simulink library "Tower"  (Simulink 7.9)
settings: Solver=ode45  StartTime=0.0  StopTime=10.0  RelTol=1e-3
undefined symbols (not defined in the file): WT_Params
libraries: mblibv1 x3
Description:
  | Copyright 2011 MathWorks, Inc.
settings Model: Creator=smiller  LastModifiedBy=smiller

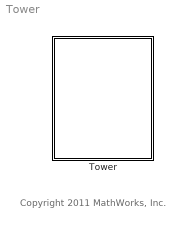
== system Tower ==
  note: Copyright 2011 MathWorks, Inc.
  Tower : Subsystem
      mask Display:
      | image(imread('Tower_IMAGE.jpg'));
      | port_label('RConn',1,'Env');
      | port_label('RConn',2,'GrVa');
      | port_label('RConn',3,'GrVb');
      | port_label('RConn',4,'GrVc');
      | port_label('LConn',1,'N');
      | port_label('LConn',2,'GrVa');
      | port_label('LConn',3,'GrVb');
      | port_label('LConn',4,'GrVc');

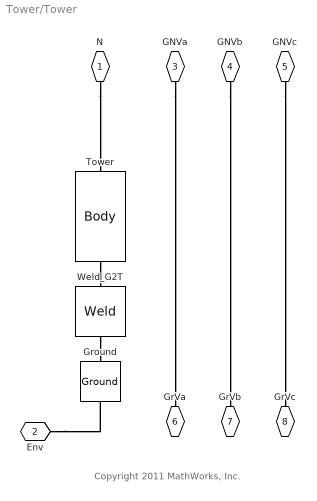
== system Tower/Tower ==
  note: Copyright 2011 MathWorks, Inc.
  Ground : mblibv1/Bodies/Ground  UpdateFromCAD=off  LeftPortType=env  RightPortType=workingframe  PhysicalDomain=Mechanical  DialogClass=GroundBlock  CoordPosition=[0 0 0]  CoordPositionUnits=m  StateVectorMgrId=-1  MachineId=[0 0]  ShowEnvPort=on
  Tower : mblibv1/Bodies/Body  LConnTagsString=CS1  RConnTagsString=CS2  UpdateFromCAD=off  DialogClass=MechanicalBodyBlock  Mass=WT_Params.Tower.mass  MassUnits=kg  InertiaUnits=kg*m^2  Inertia=WT_Params.Tower.inertia  Shape=Cylinder  ShapeDims=[1 1]  ShapeUnits=m  ShapeUse=false  Density=1  DensityUnits=kg/m^3  DensityUse=false  GraphicsMode=MACHINE_DEFAULT  BodyColorSelMode=COLORPALETTE  BodyColor=[1 1 1]  AttachedToCS=CG  CG=Left$CG$[0 0 0]$CS1$CS1$m$[0 0 0]$Euler X-Y-Z$deg$ADJOINING$false$none  WorkingFrames=Left$CS1$[0 0 0]$Adjoining$Adjoining$m$[0 0 0]$Euler X-Y-Z$deg$CG$true$none#Right$CS2$[0 WT_Params.Tower.height 0]$CS1$CS1$m$[0 0 0]$Euler X-Y-Z$deg$CG$true$none#Right$CS5$[0 0 0]$CG$CG$m$[0 0 0]$Euler X-Y-Z$deg$CG$false$none#Right$CS7$[WT_Params.Tower.base_radius*cos(0) 0 WT_Params.Tower.base_radius*sin(0)]$CG$CG$m$[0 0 0]$Euler X-Y-Z$deg$CG$false$none#Right$CS8$[WT_Params.Tower.base_radius*cos(0.2*pi) 0 WT_Params.Tower.base_radius*sin(0.2*pi)]$CG$CG$m$[0 0 0]$Euler X-Y-Z$deg$CG$false$none#Right$CS9$[WT_Params.Tower.base_radius*cos(0.4*pi) 0 WT_Params.Tower.base_radius*sin(0.4*pi)]$CG$CG$m$[0 0 0]$Euler X-Y-Z$deg$CG$false$none#Right$CS10$[WT_Params.Tower.base_radius*cos(0.6*pi) 0 WT_Params.Tower.base_radius*sin(0.6*pi)]$CG$CG$m$[0 0 0]$Euler X-Y-Z$deg$CG$false$none#Right$CS11$[WT_Params.Tower.base_radius*cos(0.8*pi) 0 WT_Params.Tower.base_radius*sin(0.8*pi)]$CG$CG$m$[0 0 0]$Euler X-Y-Z$deg$CG$false$none#Right$CS12$[WT_Params.Tower.base_radius*cos(1.0*pi) 0 WT_Params.Tower.base_radius*sin(1.0*pi)]$CG$CG$m$[0 0 0]$Euler X-Y-Z$deg$CG$false$none#Right$CS13$[WT_Params.Tower.base_radius*cos(1.2*pi) 0 WT_Params.Tower.base_radius*sin(1.2*pi)]$CG$CG$m$[0 0 0]$Euler X-Y-Z$deg$CG$false$none#Right$CS14$[WT_Params.Tower.base_radius*cos(1.4*pi) 0 WT_Params.Tower.base_radius*sin(1.4*pi)]$CG$CG$m$[0 0 0]$Euler X-Y-Z$deg$CG$false$none#Right$CS15$[WT_Params.Tower.base_radius*cos(1.6*pi) 0 WT_Params.Tower.base_radius*sin(1.6*pi)]$CG$CG$m$[0 0 0]$Euler X-Y-Z$deg$CG$false$none#Right$CS16$[WT_Params.Tower.base_radius*cos(1.8*pi) 0 WT_Params.Tower.base_radius*sin(1.8*pi)]$CG$CG$m$[0 0 0]$Euler X-Y-Z$deg$CG$false$none#Right$CS17$[WT_Params.Tower.top_radius*cos(0) WT_Params.Tower.height WT_Params.Tower.top_radius*sin(0)]$CG$CG$m$[0 0 0]$Euler X-Y-Z$deg$CG$false$none#Right$CS18$[WT_Params.Tower.top_radius*cos(0.2*pi) WT_Params.Tower.height WT_Params.Tower.top_radius*sin(0.2*pi)]$CG$CG$m$[0 0 0]$Euler X-Y-Z$deg$CG$false$none#Right$CS19$[WT_Params.Tower.top_radius*cos(0.4*pi) WT_Params.Tower.height WT_Params.Tower.top_radius*sin(0.4*pi)]$CG$CG$m$[0 0 0]$Euler X-Y-Z$deg$CG$false$none#Right$CS20$[WT_Params.Tower.top_radius*cos(0.6*pi) WT_Params.Tower.height WT_Params.Tower.top_radius*sin(0.6*pi)]$CG$CG$m$[0 0 0]$Euler X-Y-Z$deg$CG$false$none#Right$CS21$[WT_Params.Tower.top_radius*cos(0.8*pi) WT_Params.Tower.height WT_Params.Tower.top_radius*sin(0.8*pi)]$CG$CG$m$[0 0 0]$Euler X-Y-Z$deg$CG$false$none#Right$CS22$[WT_Params.Tower.top_radius*cos(1.0*pi) WT_Params.Tower.height WT_Params.Tower.top_radius*sin(1.0*pi)]$CG$CG$m$[0 0 0]$Euler X-Y-Z$deg$CG$false$none#Right$CS23$[WT_Params.Tower.top_radius*cos(1.2*pi) WT_Params.Tower.height WT_Params.Tower.top_radius*sin(1.2*pi)]$CG$CG$m$[0 0 0]$Euler X-Y-Z$deg$CG$false$none#Right$CS24$[WT_Params.Tower.top_radius*cos(1.4*pi) WT_Params.Tower.height WT_Params.Tower.top_radius*sin(1.4*pi)]$CG$CG$m$[0 0 0]$Euler X-Y-Z$deg$CG$false$none#Right$CS25$[WT_Params.Tower.top_radius*cos(1.6*pi) WT_Params.Tower.height WT_Params.Tower.top_radius*sin(1.6*pi)]$CG$CG$m$[0 0 0]$Euler X-Y-Z$deg$CG$false$none#Right$CS26$[WT_Params.Tower.top_radius*cos(1.8*pi) WT_Params.Tower.height WT_Params.Tower.top_radius*sin(1.8*pi)]$CG$CG$m$[0 0 0]$Euler X-Y-Z$deg$CG$false$none  CGPos=[0 0 0]  CGRot=[0 0 0]  CS0Pos=[]  CS0Rot=[]  CS1Pos=[0 0 0]  CS1Rot=[0 0 0]  CS2Pos=[0 WT_Params.Tower.height 0]  CS2Rot=[0 0 0]  CS3Pos=[]  CS3Rot=[]  CS4Pos=[]  CS4Rot=[]  CS5Pos=[0 0 0]  CS5Rot=[0 0 0]  CS6Pos=[]  CS6Rot=[]  CS7Pos=[WT_Params.Tower.base_radius*cos(0) 0 WT_Params.Tower.base_radius*sin(0)]  CS7Rot=[0 0 0]  CS8Pos=[WT_Params.Tower.base_radius*cos(0.2*pi) 0 WT_Params.Tower.base_radius*sin(0.2*pi)]  CS8Rot=[0 0 0]  CS9Pos=[WT_Params.Tower.base_radius*cos(0.4*pi) 0 WT_Params.Tower.base_radius*sin(0.4*pi)]  CS9Rot=[0 0 0]  CS10Pos=[WT_Params.Tower.base_radius*cos(0.6*pi) 0 WT_Params.Tower.base_radius*sin(0.6*pi)]  CS10Rot=[0 0 0]  CS11Pos=[WT_Params.Tower.base_radius*cos(0.8*pi) 0 WT_Params.Tower.base_radius*sin(0.8*pi)]  CS11Rot=[0 0 0]  CS12Pos=[WT_Params.Tower.base_radius*cos(1.0*pi) 0 WT_Params.Tower.base_radius*sin(1.0*pi)]  CS12Rot=[0 0 0]  CS13Pos=[WT_Params.Tower.base_radius*cos(1.2*pi) 0 WT_Params.Tower.base_radius*sin(1.2*pi)]  CS13Rot=[0 0 0]  CS14Pos=[WT_Params.Tower.base_radius*cos(1.4*pi) 0 WT_Params.Tower.base_radius*sin(1.4*pi)]  CS14Rot=[0 0 0]  CS15Pos=[WT_Params.Tower.base_radius*cos(1.6*pi) 0 WT_Params.Tower.base_radius*sin(1.6*pi)]  CS15Rot=[0 0 0]  CS16Pos=[WT_Params.Tower.base_radius*cos(1.8*pi) 0 WT_Params.Tower.base_radius*sin(1.8*pi)]  CS16Rot=[0 0 0]  CS17Pos=[WT_Params.Tower.top_radius*cos(0) WT_Params.Tower.height WT_Params.Tower.top_radius*sin(0)]  CS17Rot=[0 0 0]  CS18Pos=[WT_Params.Tower.top_radius*cos(0.2*pi) WT_Params.Tower.height WT_Params.Tower.top_radius*sin(0.2*pi)]  CS18Rot=[0 0 0]  CS19Pos=[WT_Params.Tower.top_radius*cos(0.4*pi) WT_Params.Tower.height WT_Params.Tower.top_radius*sin(0.4*pi)]  CS19Rot=[0 0 0]  CS20Pos=[WT_Params.Tower.top_radius*cos(0.6*pi) WT_Params.Tower.height WT_Params.Tower.top_radius*sin(0.6*pi)]  CS20Rot=[0 0 0]
  Weld_G2T : mblibv1/Joints/Weld  PhysicalDomain=mechanical  SubClassName=Unknown  LeftPortType=blob  RightPortType=blob  LConnTagsString=__newl0  RConnTagsString=__newr0  UpdateFromCAD=off  NumSAPorts=0  CutJoint=off  MarkAsCut=off  Primitives=weld  PrimitiveProps=W$WORLD$[0 0 0]$weld  DialogClass=JointBlock  WAxis=[0 0 0]
  N : PMIOPort  Port=1  Side=Left
  Env : PMIOPort  Port=2  Side=Right
  GNVa : PMIOPort  Tag=PMCPort  Port=3  Side=Left
  GNVb : PMIOPort  Tag=PMCPort  Port=4  Side=Left
  GNVc : PMIOPort  Tag=PMCPort  Port=5  Side=Left
  GrVa : PMIOPort  Tag=PMCPort  Port=6  Side=Right
  GrVb : PMIOPort  Tag=PMCPort  Port=7  Side=Right
  GrVc : PMIOPort  Tag=PMCPort  Port=8  Side=Right
  connections:
  Weld_G2T/RConn1 -- Ground/RConn1
  Tower/LConn1 -- Weld_G2T/LConn1
  N/RConn1 -- Tower/RConn1
  Env/RConn1 -- Ground/LConn1
  GNVa/RConn1 -- GrVa/RConn1
  GNVb/RConn1 -- GrVb/RConn1
  GNVc/RConn1 -- GrVc/RConn1
